simulink library "CarModelLibrary"  (R2023b)
settings: Solver=VariableStepAuto  StartTime=0.0  StopTime=10.0  RelTol=1e-3
libraries: simulink x6
settings Model: Creator=arturogonzalez  LastModifiedBy=franc
settings SolverCC: AlgebraicLoopSolver=TrustRegion
settings DebuggingCC: UnconnectedInputMsg=warning  UnconnectedOutputMsg=warning  UnconnectedLineMsg=warning
settings ModelReferenceCC: EnableRefExpFcnMdlSchedulingChecks=on

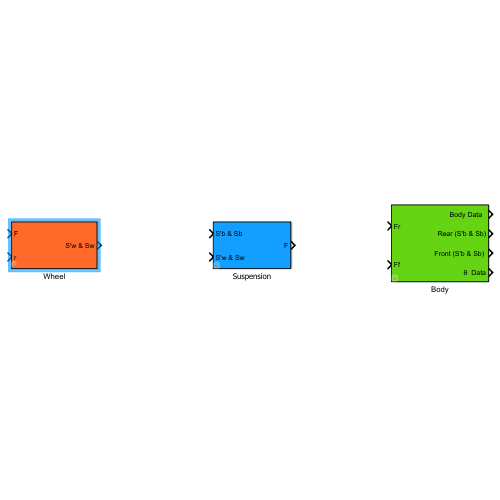
[thumbnail: Simulink's stored preview of the top-level diagram]
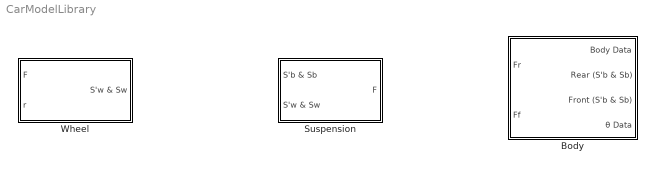
== system CarModelLibrary ==
  Body : Subsystem  mask{mb=700, I=650, a=1.35, b=1.5, g=9.81}
      mask prompts: mb "Body Mass"; I "Body Inertia"; a "Front tyre distance from CoG"; b "Rear tyre distance from CoG"; g "Gravitational acceleration"
  Suspension : Subsystem  mask{ks=2e4, ksstiff=20, x0=0.2, csb=600, csr=1200}
      mask prompts: ks "Spring Stiffness (N/m)"; ksstiff "Spring Hardening (ks)"; x0 "Spring Hardening (x0)"; csb "Bump Damping Rate (Ns/m)"; csr "Rebound Damping Rate (Ns/m)"
  Wheel : Subsystem  mask{mw=20, Kt=14e4, g=9.81}
      mask prompts: mw "Wheel Mass (Kg)"; Kt "Tyre Stiffness"; g "Gravitational acceleration"

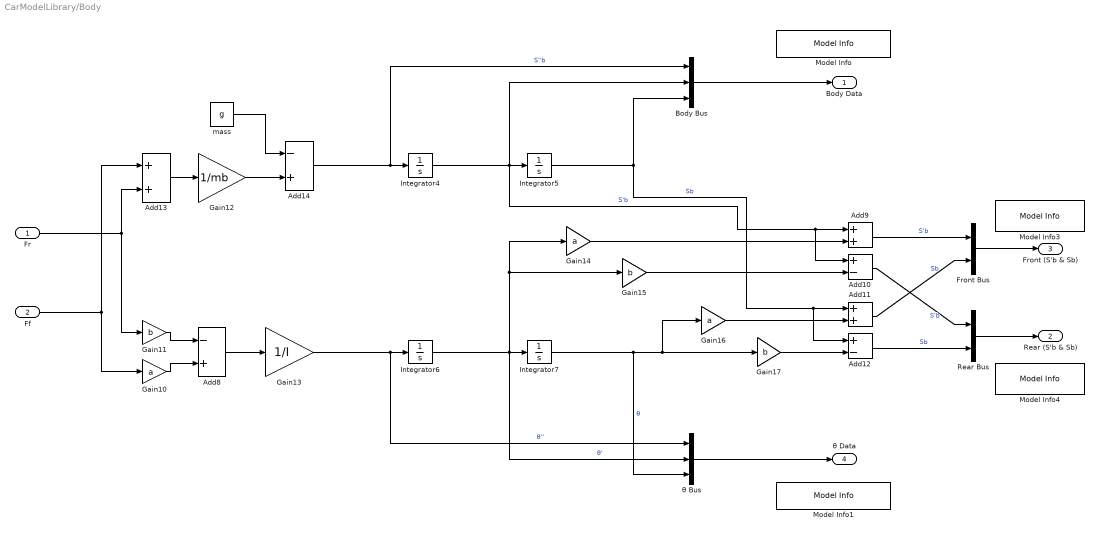
== system CarModelLibrary/Body ==
  Fr : Inport
  Ff : Inport  Port=2
  Add10 : Sum  Inputs=+-
  Add11 : Sum
  Add12 : Sum  Inputs=+-
  Add13 : Sum
  Add14 : Sum  Inputs=-+
  Add8 : Sum  Inputs=-+
  Add9 : Sum
  Body Bus : BusCreator  Inputs=3
  Front Bus : BusCreator  Inputs=2
  Gain10 : Gain  Gain=a
  Gain11 : Gain  Gain=b
  Gain12 : Gain  Gain=1/mb
  Gain13 : Gain  Gain=1/I
  Gain14 : Gain  Gain=a
  Gain15 : Gain  Gain=b
  Gain16 : Gain  Gain=a
  Gain17 : Gain  Gain=b
  Integrator{4..7} (4 alike) : Integrator
  Model Info : simulink/Model-Wide Utilities/Model Info  Frame=on  DisplayStringWithTags=mb*S''b = Ff + Fr - mb*g  HorizontalTextAlignment=Center  LeftAlignmentValue=0.5
  Model Info1 : simulink/Model-Wide Utilities/Model Info  Frame=on  DisplayStringWithTags=I*θ'' = a*Ff - b*Fr  HorizontalTextAlignment=Center  LeftAlignmentValue=0.5
  Model Info3 : simulink/Model-Wide Utilities/Model Info  Frame=on  DisplayStringWithTags=|  HorizontalTextAlignment=Center  LeftAlignmentValue=0.5
      | S'bf = S'b + a*θ'
      | Sbf = Sb + a*θ
  Model Info4 : simulink/Model-Wide Utilities/Model Info  Frame=on  DisplayStringWithTags=|  HorizontalTextAlignment=Center  LeftAlignmentValue=0.5
      | S'br = S'b - b*θ'
      | Sbr = Sb - b*θ
  Rear Bus : BusCreator  Inputs=2
  mass : Constant  Value=g
  θ Bus : BusCreator  Inputs=3
  "Body Data " : Outport
  Rear (S'b & Sb) : Outport  Port=2
  "Front (S'b & Sb) " : Outport  Port=3
  θ Data : Outport  Port=4
  wires:
  Body Bus/1 -> "Body Data "/1
  Integrator6/1 -> θ Bus/2, Integrator7/1, Gain14/1, Gain15/1  "θ'"
  Integrator4/1 -> Body Bus/2, Add9/1, Add10/1, Integrator5/1  "S'b"
  Ff/1 -> Gain10/1, Add13/1
  Gain14/1 -> Add9/2
  Integrator7/1 -> θ Bus/3, Gain17/1, Gain16/1  "θ"
  Gain11/1 -> Add8/1
  Fr/1 -> Add13/2, Gain11/1
  Add12/1 -> Rear Bus/2  "Sb"
  Gain15/1 -> Add10/2
  θ Bus/1 -> θ Data/1
  Add11/1 -> Front Bus/2  "Sb"
  Add9/1 -> Front Bus/1  "S'b"
  Gain16/1 -> Add11/2
  Add8/1 -> Gain13/1
  Front Bus/1 -> "Front (S'b & Sb) "/1
  Integrator5/1 -> Body Bus/3, Add11/1, Add12/1  "Sb"
  Add14/1 -> Body Bus/1, Integrator4/1  "S''b"
  Rear Bus/1 -> Rear (S'b & Sb)/1
  Gain17/1 -> Add12/2
  mass/1 -> Add14/1
  Add10/1 -> Rear Bus/1  "S'b"
  Add13/1 -> Gain12/1
  Gain13/1 -> θ Bus/1, Integrator6/1  "θ''"
  Gain10/1 -> Add8/2
  Gain12/1 -> Add14/2

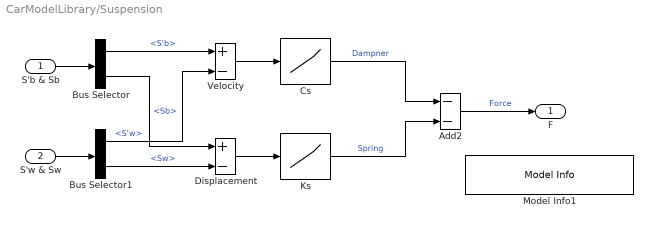
== system CarModelLibrary/Suspension ==
  S'b & Sb : Inport
  S'w & Sw : Inport  Port=2
  Add2 : Sum  Inputs=--
  Bus Selector : BusSelector  OutputSignals=S'b,Sb
  Bus Selector1 : BusSelector  OutputSignals=S'w,Sw
  Cs : Lookup_n-D  NumberOfTableDimensions=1  BreakpointsForDimension1=[-1, 0, 1]  Table=[-csr, 0, csb]  InternalRulePriority=Speed  RndMeth=Simplest
  Displacement : Sum  Inputs=+-
  Ks : Lookup_n-D  NumberOfTableDimensions=1  BreakpointsForDimension1=[-2*x0, -x0, x0, 2*x0]  Table=[-(ks+ksstiff*ks)*x0, -ks*x0, ks*x0, (ks+ksstiff*ks)*x0]  InternalRulePriority=Speed  RndMeth=Simplest
  Model Info1 : simulink/Model-Wide Utilities/Model Info  Frame=on  DisplayStringWithTags="F = -Ks (Sb - Sw) - Cs (S'b  - S'w)"  HorizontalTextAlignment=Center  LeftAlignmentValue=0.5
  Velocity : Sum  Inputs=+-
  F : Outport
  wires:
  S'w & Sw/1 -> Bus Selector1/1
  Bus Selector1/2 -> Displacement/2  "<Sw>"
  Add2/1 -> F/1  "Force"
  S'b & Sb/1 -> Bus Selector/1
  Bus Selector1/1 -> Velocity/2  "<S'w>"
  Bus Selector/1 -> Velocity/1  "<S'b>"
  Bus Selector/2 -> Displacement/1  "<Sb>"
  Displacement/1 -> Ks/1
  Velocity/1 -> Cs/1
  Cs/1 -> Add2/1  "Dampner"
  Ks/1 -> Add2/2  "Spring"

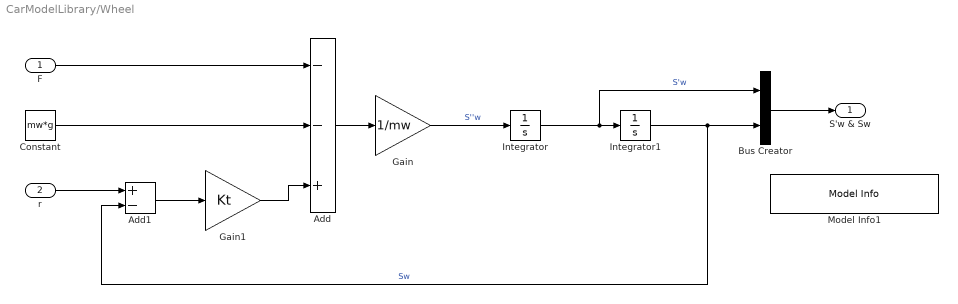
== system CarModelLibrary/Wheel ==
  F : Inport
  r : Inport  Port=2
  Add : Sum  Inputs=--+
  Add1 : Sum  Inputs=+-
  Bus Creator : BusCreator  Inputs=2
  Constant : Constant  Value=mw*g
  Gain : Gain  Gain=1/mw
  Gain1 : Gain  Gain=Kt
  Integrator : Integrator
  Integrator1 : Integrator
  Model Info1 : simulink/Model-Wide Utilities/Model Info  Frame=on  DisplayStringWithTags=m * S''w = -F + Kt (r-S) - m*g  HorizontalTextAlignment=Center  LeftAlignmentValue=0.5
  S'w & Sw : Outport
  wires:
  r/1 -> Add1/1
  Add1/1 -> Gain1/1
  Integrator/1 -> Bus Creator/1, Integrator1/1  "S'w"
  Bus Creator/1 -> S'w & Sw/1
  Integrator1/1 -> Bus Creator/2, Add1/2  "Sw"
  Add/1 -> Gain/1
  Gain/1 -> Integrator/1  "S''w"
  Constant/1 -> Add/2
  F/1 -> Add/1
  Gain1/1 -> Add/3
